simulink model "MotorSoftStartModel"  (R2025a)
settings: Solver=VariableStepAuto  StartTime=0.0  StopTime=10.0  RelTol=1e-3
libraries: simulink x1
settings Model: Creator=mahij  LastModifiedBy=mahij

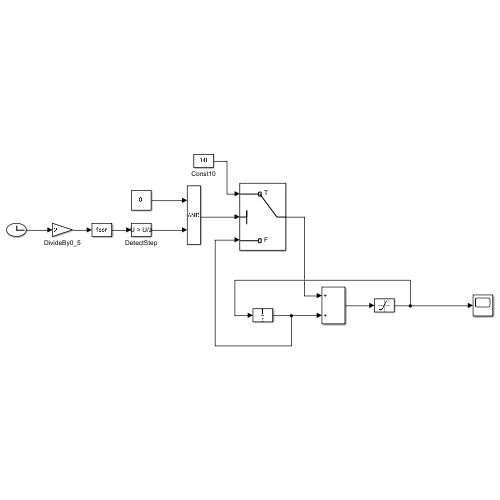
[thumbnail: Simulink's stored preview of the top-level diagram]
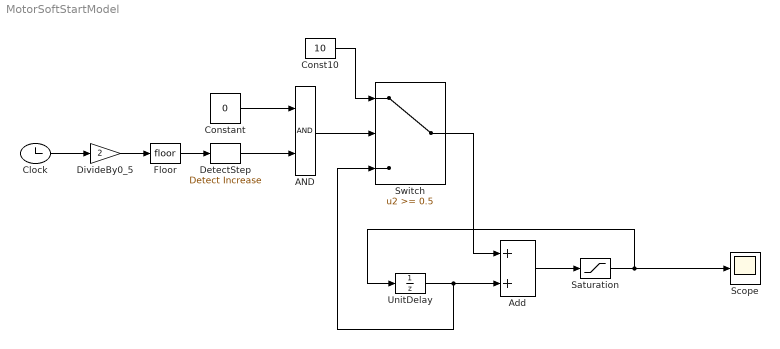
== system MotorSoftStartModel ==
  AND : Logic  AllPortsSameDT=off  OutDataTypeStr=boolean
  Add : Sum
  Clock : Clock
  Const10 : Constant  Value=10
  Constant : Constant  Value=0
  DetectStep : simulink/Logic and Bit Operations/Detect Increase  vinit=0.0  OutDataTypeStr=boolean
  DivideBy0_5 : Gain  Gain=2
  Floor : Rounding
  Saturation : Saturate  UpperLimit=100  LowerLimit=0
  Scope : Scope
      settings: ActiveDisplayYMinimum=-12.499999999999996  ActiveDisplayYMaximum=112.5
  Switch : Switch  Threshold=0.5  SaturateOnIntegerOverflow=off  InputSameDT=off
  UnitDelay : UnitDelay  SampleTime=0.5  HasFrameUpgradeWarning=on
  wires:
  Constant/1 -> AND/1
  Clock/1 -> DivideBy0_5/1
  DivideBy0_5/1 -> Floor/1
  Floor/1 -> DetectStep/1
  DetectStep/1 -> AND/2
  AND/1 -> Switch/2
  Const10/1 -> Switch/1
  UnitDelay/1 -> Switch/3, Add/2
  Switch/1 -> Add/1
  Add/1 -> Saturation/1
  Saturation/1 -> UnitDelay/1, Scope/1
